simulink model "Lab1_6D"  (R2018a)
settings: Solver=VariableStepAuto  StartTime=0.0  StopTime=90  RelTol=1e-6
settings Model: Creator=melab2  LastModifiedBy=rahul

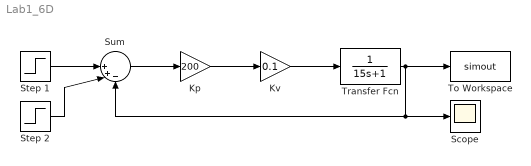
== system Lab1_6D ==
  Kp : Gain  Gain=200
  Kv : Gain  Gain=0.1
  Scope : Scope
  "Step 1 " : Step  SampleTime=0
  Step 2 : Step  Time=75  After=-2  SampleTime=0
  Sum : Sum  Inputs=||++-
  To Workspace : ToWorkspace  VariableName=simout  SampleTime=-1
  Transfer Fcn : TransferFcn  Denominator=[15 1]
  wires:
  Sum/1 -> Kp/1
  Kp/1 -> Kv/1
  Kv/1 -> Transfer Fcn/1
  Transfer Fcn/1 -> Sum/3, Scope/1, To Workspace/1
  "Step 1 "/1 -> Sum/1
  Step 2/1 -> Sum/2
